simulink model "MATLAB_TEST"  (R2019b)
settings: Solver=FixedStepDiscrete  StartTime=0  StopTime=50  FixedStep=0.0025  RelTol=1e-3
undefined symbols (not defined in the file): BCM_COM_PROC_P20, BCM_COM_PROC_P20_SFW_R2018b, BCM_COM_PROC_P2_5, BCM_COM_PROC_P2_5_SFW_R2018b, BCM_COM_PROC_P5, BCM_COM_PROC_P5_SFW_R2018b, BCMA_ACCU_PT_Conf_Flt, BCMA_ACCU_PT_Unconf_Flt, BCMA_Antiskid_Off_Sanction, BCMA_Avionics_Conf_Flt, BCMA_BCM_CCDL_Conf_Flt, BCMA_BCM_CCDL_Unconf_Flt, BCMA_BCM_DBCU_INHIBITION_Conf_Flt, BCMA_BCM_DBCU_INHIBITION_Unconf_Flt, BCMA_BCP_ALT_Disp_Sw_Conf_Flt, BCMA_BCP_ALT_Disp_Sw_Unconf_Flt, BCMA_BCP_ALT_SW_ON_CMD_Conf_Flt, BCMA_BCP_ALT_SW_ON_CMD_Unconf_Flt, BCMA_BCP_PARK_OFF_SW_CMD_Conf_Flt, BCMA_BCP_PARK_OFF_SW_CMD_Unconf_Flt, BCMA_CF_BSELV_JCL, BCMA_CF_BSELV_JOP, BCMA_CF_BSELV_OC, BCMA_CF_BSELV_SC, BCMA_CF_LH_SV_JCL, BCMA_CF_LH_SV_JOP, BCMA_CF_LH_SV_OC, BCMA_CF_LH_SV_SC, BCMA_CF_PARK_BRK, BCMA_CF_RESIDUAL_PRESS, BCMA_CF_RH_SV_JCL, BCMA_CF_RH_SV_JOP, BCMA_CF_RH_SV_OC, BCMA_CF_RH_SV_SC, BCMA_CF_SELV_JCL, BCMA_CF_SELV_JOP, BCMA_CF_SELV_OC, BCMA_CF_SELV_SC, BCMA_CF_SV_DRIFT, BCMA_DBCU_ALT_MODE_Conf_Flt, BCMA_DBCU_ALT_MODE_Unconf_Flt, BCMA_DBCU_BRK_ORDER_FAIL_Conf_Flt, BCMA_DBCU_BRK_ORDER_FAIL_Unconf_Flt, BCMA_DBCU_Conf_Flt, BCMA_DBCU_DISPATCH_SW_ON_Conf_Flt, BCMA_DBCU_DISPATCH_SW_ON_Unconf_Flt, BCMA_DBCU_FAILED_Conf_Flt, BCMA_DBCU_FAILED_Unconf_Flt, BCMA_DFCS1_Capsule_Validity, BCMA_DFCS1_Label202_Corrupted, BCMA_DFCS1_Label202_Not_Refreshed, BCMA_DFCS1_Label204_Corrupted, BCMA_DFCS1_Label204_Not_Refreshed, BCMA_DFCS1_Label205_Corrupted, BCMA_DFCS1_Label205_Not_Refreshed, BCMA_DFCS1_Label206_Corrupted, BCMA_DFCS1_Label206_Not_Refreshed, BCMA_DFCS1_Label207_Corrupted, BCMA_DFCS1_Label207_Not_Refreshed, BCMA_DFCS3_Capsule_Validity ... (+762)
libraries: simulink x73, lib_MBD_Control x5
(part 7 of 16)

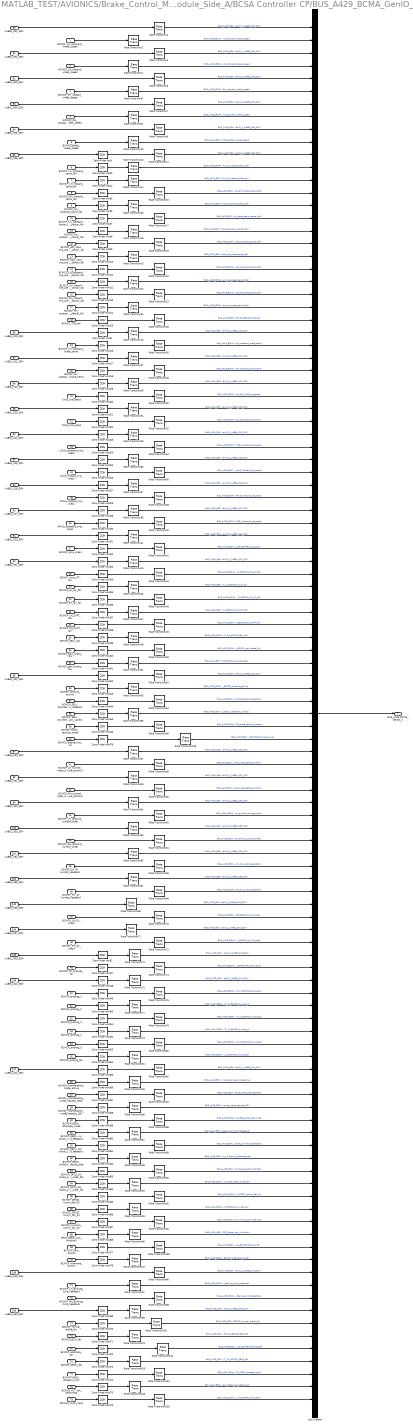
== system MATLAB_TEST/AVIONICS/Brake_Control_Module_Side_A/BCSA Controller CP/BUS_A429_BCMA_GenIO_2_TX ==
  BCMCP_LH_outboard_wheel_speed : Inport  OutDataTypeStr=single
  BCMCP_LH_inboard_wheel_speed : Inport  Port=2  OutDataTypeStr=single
  BCMCP_RH_inboard_wheel_speed : Inport  Port=3  OutDataTypeStr=single
  BCMCP_RH_outboard_wheel_speed : Inport  Port=4  OutDataTypeStr=single
  BCMCP_global_wheel_speed : Inport  Port=5  OutDataTypeStr=single
  BCMCP_LH_outboard_tacho_fail : Inport  Port=6  OutDataTypeStr=boolean
  BCMCP_LH_inboard_tacho_fail : Inport  Port=7  OutDataTypeStr=boolean
  BCMCP_RH_inboard_tacho_fail : Inport  Port=8  OutDataTypeStr=boolean
  BCMCP_RH_outboard_tacho_fail : Inport  Port=9  OutDataTypeStr=boolean
  BCMCP_LH_outboard_brake_temp_sensor_fail : Inport  Port=10  OutDataTypeStr=boolean
  BCMCP_RH_outboard_brake_temp_sensor_fail : Inport  Port=11  OutDataTypeStr=boolean
  BCMCP_left_nose_tire_press_sensor_fail : Inport  Port=12  OutDataTypeStr=boolean
  BCMCP_right_nose_tire_press_sensor_fail : Inport  Port=13  OutDataTypeStr=boolean
  BCMCP_LH_outboard_tire_press_sensor_fail : Inport  Port=14  OutDataTypeStr=boolean
  BCMCP_LH_inboard_tire_press_sensor_fail : Inport  Port=15  OutDataTypeStr=boolean
  BCMCP_RH_inboard_tire_press_sensor_fail : Inport  Port=16  OutDataTypeStr=boolean
  BCMCP_RH_outboard_tire_press_sensor_fail : Inport  Port=17  OutDataTypeStr=boolean
  BCMCP_TPIS_fail : Inport  Port=18  OutDataTypeStr=boolean
  BCMCP_LH_outboard_brake_temp : Inport  Port=19  OutDataTypeStr=single
  BCMCP_RH_outboard_brake_temp : Inport  Port=20  OutDataTypeStr=single
  LNLG_tire_press : Inport  Port=21  OutDataTypeStr=single
  RNLG_tire_press : Inport  Port=22  OutDataTypeStr=single
  LMLG_outboard_tire_press : Inport  Port=23  OutDataTypeStr=single
  LMLG_inboard_tire_press : Inport  Port=24  OutDataTypeStr=single
  RMLG_inboard_tire_press : Inport  Port=25  OutDataTypeStr=single
  RMLG_outboard_tire_press : Inport  Port=26  OutDataTypeStr=single
  BCMCP_accu_press : Inport  Port=27  OutDataTypeStr=single
  BCMCP_Accu_PT_fail : Inport  Port=28  OutDataTypeStr=boolean
  BCMCP_LH_SV_fail : Inport  Port=29  OutDataTypeStr=boolean
  BCMCP_RH_SV_fail : Inport  Port=30  OutDataTypeStr=boolean
  BCMCP_LH_SVPT_fail : Inport  Port=31  OutDataTypeStr=boolean
  BCMCP_RH_SVPT_fail : Inport  Port=32  OutDataTypeStr=boolean
  BCMCP_SELV_fail : Inport  Port=33  OutDataTypeStr=boolean
  BCMCP_park_brake_ON : Inport  Port=34  OutDataTypeStr=boolean
  BCMCP_park_brake_fail : Inport  Port=35  OutDataTypeStr=boolean
  BCMCP_antiskid_activity : Inport  Port=36  OutDataTypeStr=boolean
  BCMCP_SELV_discrete_status_readback : Inport  Port=37  OutDataTypeStr=boolean
  BCMCP_SELV_discrete_status_readback_validity : Inport  Port=38  OutDataTypeStr=boolean
  BCMCP_brake_residual_press : Inport  Port=39  OutDataTypeStr=boolean
  BCMCP_Engine_Run_Up : Inport  Port=40  OutDataTypeStr=boolean
  BCMCP_LH_current_order_before_antiskid : Inport  Port=41  OutDataTypeStr=single
  BCMCP_RH_current_order_before_antiskid : Inport  Port=42  OutDataTypeStr=single
  BCMCP_LH_antiskid_current_order : Inport  Port=43  OutDataTypeStr=single
  BCMCP_RH_antiskid_current_order : Inport  Port=44  OutDataTypeStr=single
  BCMCP_LH_SV_current_readback : Inport  Port=45  OutDataTypeStr=single
  BCMCP_RH_SV_current_readback : Inport  Port=46  OutDataTypeStr=single
  BCMCP_LH_SV_press : Inport  Port=47  OutDataTypeStr=single
  BCMCP_RH_SV_press : Inport  Port=48  OutDataTypeStr=single
  BCMCP_PP_channel_ID : Inport  Port=49
  BCMCP_pinprog_1 : Inport  Port=50  OutDataTypeStr=boolean
  BCMCP_pinprog_2 : Inport  Port=51  OutDataTypeStr=boolean
  BCMCP_pinprog_3 : Inport  Port=52  OutDataTypeStr=boolean
  BCMCP_pinprog_4 : Inport  Port=53  OutDataTypeStr=boolean
  BCMCP_pinprog_5 : Inport  Port=54  OutDataTypeStr=boolean
  BCMCP_pinprog_fail : Inport  Port=55  OutDataTypeStr=boolean
  BCMCP_maintenance_mode_active : Inport  Port=56  OutDataTypeStr=boolean
  BCMCP_maintenance_mode_request_GND : Inport  Port=57  OutDataTypeStr=boolean
  BCMCP_maintenance_mode_request_28V : Inport  Port=58  OutDataTypeStr=boolean
  BCMCP_DBCU_alternate_mode : Inport  Port=59  OutDataTypeStr=boolean
  BCMCP_DBCU_LH_brake_command_feedback : Inport  Port=60  OutDataTypeStr=boolean
  BCMCP_DBCU_RH_brake_command_feedback : Inport  Port=61  OutDataTypeStr=boolean
  BCMCP_DBCU_inhibition_opposite_side : Inport  Port=62  OutDataTypeStr=boolean
  BCMCP_DFCS_LH_brake_pedal_order_fail : Inport  Port=63  OutDataTypeStr=boolean
  BCMCP_DFCS_RH_brake_pedal_order_fail : Inport  Port=64  OutDataTypeStr=boolean
  BCMCP_DFCS1_comm_fail_RX : Inport  Port=65  OutDataTypeStr=boolean
  BCMCP_DFCS2_comm_fail_RX : Inport  Port=66  OutDataTypeStr=boolean
  BCMCP_Avionics_comm_fail_RX : Inport  Port=67  OutDataTypeStr=boolean
  DFCS_Decel_Law_Inhibition : Inport  Port=68  OutDataTypeStr=boolean
  BCMCP_Park_Switch : Inport  Port=69  OutDataTypeStr=boolean
  BCMCP_Alternate_Switch : Inport  Port=70  OutDataTypeStr=boolean
  BCMCP_LH_Braking_Cmd_Feedback : Inport  Port=71  OutDataTypeStr=single
  BCMCP_RH_Braking_Cmd_Feedback : Inport  Port=72  OutDataTypeStr=single
  BCMCP_normal_brake_fail : Inport  Port=73  OutDataTypeStr=boolean
  BCMCP_BCM_fail : Inport  Port=74  OutDataTypeStr=boolean
  BCMCP_alternate_fail : Inport  Port=75  OutDataTypeStr=boolean
  BCMCP_DBCU_fail : Inport  Port=76  OutDataTypeStr=boolean
  BCMCP_DBCU_dispatch_conf : Inport  Port=77  OutDataTypeStr=boolean
  BCMCP_PLT_not_performed : Inport  Port=78  OutDataTypeStr=boolean
  BCMCP_Minor_Fault : Inport  Port=79  OutDataTypeStr=boolean
  LABEL_001_SSM : Inport  Port=80
  LABEL_002_SSM : Inport  Port=81
  LABEL_003_SSM : Inport  Port=82
  LABEL_004_SSM : Inport  Port=83
  LABEL_005_SSM : Inport  Port=84
  LABEL_006_SSM : Inport  Port=85
  LABEL_010_SSM : Inport  Port=86
  LABEL_011_SSM : Inport  Port=87
  LABEL_012_SSM : Inport  Port=88
  LABEL_013_SSM : Inport  Port=89
  LABEL_014_SSM : Inport  Port=90
  LABEL_015_SSM : Inport  Port=91
  LABEL_016_SSM : Inport  Port=92
  LABEL_017_SSM : Inport  Port=93
  LABEL_020_SSM : Inport  Port=94
  LABEL_021_SSM : Inport  Port=95
  LABEL_022_SSM : Inport  Port=96
  LABEL_030_SSM : Inport  Port=97
  LABEL_031_SSM : Inport  Port=98
  LABEL_032_SSM : Inport  Port=99
  LABEL_033_SSM : Inport  Port=100
  LABEL_034_SSM : Inport  Port=101
  LABEL_035_SSM : Inport  Port=102
  LABEL_036_SSM : Inport  Port=103
  LABEL_037_SSM : Inport  Port=104
  LABEL_040_SSM : Inport  Port=105
  LABEL_041_SSM : Inport  Port=106
  LABEL_042_SSM : Inport  Port=107
  LABEL_043_SSM : Inport  Port=108
  LABEL_050_SSM : Inport  Port=109
  Bus Creator : BusCreator  Inputs=109  OutDataTypeStr=Bus: SMLK_BUS_A429_BCMA_GenIO_2  NonVirtualBus=on
      settings: InheritFromInputs=off
  Rate Transition{1..109} (109 alike) : RateTransition  Deterministic=off  OutPortSampleTime=1/50
      settings: AttributesFormatString=OutPortSampleTime %<OutPortSampleTime>
  Zero-Order Hold{,3..15,31..46,55..79} (55 alike) : ZeroOrderHold  SampleTime=0.08
      settings: AttributesFormatString=SampleTime %<SampleTime>
  Zero-Order Hold{1,16..30} (16 alike) : ZeroOrderHold  SampleTime=0.32
      settings: AttributesFormatString=SampleTime %<SampleTime>
  Zero-Order Hold{2,47..54} (9 alike) : ZeroOrderHold  SampleTime=1.28
      settings: AttributesFormatString=SampleTime %<SampleTime>
  BUS_A429_BCMA_GenIO_2 : Outport  VectorParamsAs1DForOutWhenUnconnected=off
  wires:
  Rate Transition34/1 -> Bus Creator/34  "BUS_A429_BCMA_GenIO_2_LABEL_014_LMLG_outboard_tire_press"
  Rate Transition33/1 -> Bus Creator/33  "BUS_A429_BCMA_GenIO_2_LABEL_014_SSM"
  Rate Transition35/1 -> Bus Creator/35  "BUS_A429_BCMA_GenIO_2_LABEL_015_SSM"
  Rate Transition36/1 -> Bus Creator/36  "BUS_A429_BCMA_GenIO_2_LABEL_015_LMLG_inboard_tire_press"
  Rate Transition37/1 -> Bus Creator/37  "BUS_A429_BCMA_GenIO_2_LABEL_016_SSM"
  Rate Transition38/1 -> Bus Creator/38  "BUS_A429_BCMA_GenIO_2_LABEL_016_RMLG_inboard_tire_press"
  Rate Transition32/1 -> Bus Creator/32  "BUS_A429_BCMA_GenIO_2_LABEL_013_RNLG_tire_press"
  Rate Transition39/1 -> Bus Creator/39  "BUS_A429_BCMA_GenIO_2_LABEL_017_SSM"
  Rate Transition11/1 -> Bus Creator/11  "BUS_A429_BCMA_GenIO_2_LABEL_006_SSM"
  Rate Transition14/1 -> Bus Creator/13  "BUS_A429_BCMA_GenIO_2_LABEL_006_DATA_BIT_12_BCMCP_LH_inboard_tacho_fail"
  Rate Transition30/1 -> Bus Creator/30  "BUS_A429_BCMA_GenIO_2_LABEL_012_LNLG_tire_press"
  Rate Transition40/1 -> Bus Creator/40  "BUS_A429_BCMA_GenIO_2_LABEL_017_RMLG_outboard_tire_press"
  Rate Transition15/1 -> Bus Creator/14  "BUS_A429_BCMA_GenIO_2_LABEL_006_DATA_BIT_13_BCMCP_RH_inboard_tacho_fail"
  Rate Transition16/1 -> Bus Creator/15  "BUS_A429_BCMA_GenIO_2_LABEL_006_DATA_BIT_14_BCMCP_RH_outboard_tacho_fail"
  Rate Transition17/1 -> Bus Creator/16  "BUS_A429_BCMA_GenIO_2_LABEL_006_DATA_BIT_15_BCMCP_LH_outboard_brake_temp_sensor_fail"
  Rate Transition29/1 -> Bus Creator/29  "BUS_A429_BCMA_GenIO_2_LABEL_012_SSM"
  Rate Transition28/1 -> Bus Creator/28  "BUS_A429_BCMA_GenIO_2_LABEL_011_BCMCP_RH_outboard_brake_temp"
  Rate Transition19/1 -> Bus Creator/18  "BUS_A429_BCMA_GenIO_2_LABEL_006_DATA_BIT_17_BCMCP_left_nose_tire_press_sensor_fail"
  Rate Transition20/1 -> Bus Creator/19  "BUS_A429_BCMA_GenIO_2_LABEL_006_DATA_BIT_18_BCMCP_right_nose_tire_press_sensor_fail"
  Rate Transition55/1 -> Bus Creator/55  "BUS_A429_BCMA_GenIO_2_LABEL_022_DATA_BIT_13_BCMCP_SELV_discrete_status_readback_validity"
  Rate Transition56/1 -> Bus Creator/56  "BUS_A429_BCMA_GenIO_2_LABEL_022_DATA_BIT_14_BCMCP_brake_residual_press"
  Rate Transition10/1 -> Bus Creator/10  "BUS_A429_BCMA_GenIO_2_LABEL_005_BCMCP_global_wheel_speed"
  Rate Transition21/1 -> Bus Creator/20  "BUS_A429_BCMA_GenIO_2_LABEL_006_DATA_BIT_19_BCMCP_LH_outboard_tire_press_sensor_fail"
  Rate Transition27/1 -> Bus Creator/27  "BUS_A429_BCMA_GenIO_2_LABEL_011_SSM"
  Rate Transition41/1 -> Bus Creator/41  "BUS_A429_BCMA_GenIO_2_LABEL_020_SSM"
  Rate Transition50/1 -> Bus Creator/50  "BUS_A429_BCMA_GenIO_2_LABEL_021_DATA_BIT_17_BCMCP_park_brake_ON"
  Rate Transition51/1 -> Bus Creator/51  "BUS_A429_BCMA_GenIO_2_LABEL_021_DATA_BIT_18_BCMCP_park_brake_fail"
  Rate Transition54/1 -> Bus Creator/54  "BUS_A429_BCMA_GenIO_2_LABEL_022_DATA_BIT_12_BCMCP_SELV_discrete_status_readback"
  Rate Transition9/1 -> Bus Creator/9  "BUS_A429_BCMA_GenIO_2_LABEL_005_SSM"
  Rate Transition42/1 -> Bus Creator/42  "BUS_A429_BCMA_GenIO_2_LABEL_020_BCMCP_accu_press"
  Rate Transition43/1 -> Bus Creator/43  "BUS_A429_BCMA_GenIO_2_LABEL_021_SSM"
  Rate Transition45/1 -> Bus Creator/45  "BUS_A429_BCMA_GenIO_2_LABEL_021_DATA_BIT_12_BCMCP_LH_SV_fail"
  Rate Transition46/1 -> Bus Creator/46  "BUS_A429_BCMA_GenIO_2_LABEL_021_DATA_BIT_13_BCMCP_RH_SV_fail"
  Rate Transition47/1 -> Bus Creator/47  "BUS_A429_BCMA_GenIO_2_LABEL_021_DATA_BIT_14_BCMCP_LH_SVPT_fail"
  Rate Transition48/1 -> Bus Creator/48  "BUS_A429_BCMA_GenIO_2_LABEL_021_DATA_BIT_15_BCMCP_RH_SVPT_fail"
  Rate Transition49/1 -> Bus Creator/49  "BUS_A429_BCMA_GenIO_2_LABEL_021_DATA_BIT_16_BCMCP_SELV_fail"
  Rate Transition26/1 -> Bus Creator/26  "BUS_A429_BCMA_GenIO_2_LABEL_010_BCMCP_LH_outboard_brake_temp"
  Rate Transition44/1 -> Bus Creator/44  "BUS_A429_BCMA_GenIO_2_LABEL_021_DATA_BIT_11_BCMCP_Accu_PT_fail"
  Rate Transition52/1 -> Bus Creator/52  "BUS_A429_BCMA_GenIO_2_LABEL_022_SSM"
  Rate Transition8/1 -> Bus Creator/8  "BUS_A429_BCMA_GenIO_2_LABEL_004_BCMCP_RH_outboard_wheel_speed"
  Rate Transition23/1 -> Bus Creator/22  "BUS_A429_BCMA_GenIO_2_LABEL_006_DATA_BIT_21_BCMCP_RH_inboard_tire_press_sensor_fail"
  Rate Transition13/1 -> Bus Creator/25  "BUS_A429_BCMA_GenIO_2_LABEL_010_SSM"
  Rate Transition53/1 -> Bus Creator/53  "BUS_A429_BCMA_GenIO_2_LABEL_022_DATA_BIT_11_BCMCP_antiskid_activity"
  Rate Transition24/1 -> Bus Creator/23  "BUS_A429_BCMA_GenIO_2_LABEL_006_DATA_BIT_22_BCMCP_RH_outboard_tire_press_sensor_fail"
  Rate Transition25/1 -> Bus Creator/24  "BUS_A429_BCMA_GenIO_2_LABEL_006_DATA_BIT_23_BCMCP_TPIS_fail"
  Rate Transition7/1 -> Bus Creator/7  "BUS_A429_BCMA_GenIO_2_LABEL_004_SSM"
  Rate Transition95/1 -> Bus Creator/96  "BUS_A429_BCMA_GenIO_2_LABEL_042_DATA_BIT_23_DFCS_Decel_Law_Inhibition"
  Rate Transition93/1 -> Bus Creator/94  "BUS_A429_BCMA_GenIO_2_LABEL_042_DATA_BIT_21_BCMCP_DFCS2_comm_fail_RX"
  Rate Transition94/1 -> Bus Creator/95  "BUS_A429_BCMA_GenIO_2_LABEL_042_DATA_BIT_22_BCMCP_Avionics_comm_fail_RX"
  Rate Transition6/1 -> Bus Creator/6  "BUS_A429_BCMA_GenIO_2_LABEL_003_BCMCP_RH_inboard_wheel_speed"
  Rate Transition92/1 -> Bus Creator/93  "BUS_A429_BCMA_GenIO_2_LABEL_042_DATA_BIT_20_BCMCP_DFCS1_comm_fail_RX"
  Rate Transition96/1 -> Bus Creator/99  "BUS_A429_BCMA_GenIO_2_LABEL_043_SSM"
  Rate Transition91/1 -> Bus Creator/92  "BUS_A429_BCMA_GenIO_2_LABEL_042_DATA_BIT_19_BCMCP_DFCS_RH_brake_pedal_order_fail"
  Rate Transition98/1 -> Bus Creator/101  "BUS_A429_BCMA_GenIO_2_LABEL_043_BCMCP_RH_Braking_Cmd_Feedback"
  Rate Transition5/1 -> Bus Creator/5  "BUS_A429_BCMA_GenIO_2_LABEL_003_SSM"
  Rate Transition90/1 -> Bus Creator/91  "BUS_A429_BCMA_GenIO_2_LABEL_042_DATA_BIT_18_BCMCP_DFCS_LH_brake_pedal_order_fail"
  Rate Transition97/1 -> Bus Creator/100  "BUS_A429_BCMA_GenIO_2_LABEL_043_BCMCP_LH_Braking_Cmd_Feedback"
  Rate Transition89/1 -> Bus Creator/90  "BUS_A429_BCMA_GenIO_2_LABEL_042_DATA_BIT_17_BCMCP_DBCU_inhibition_opposite_side"
  Rate Transition87/1 -> Bus Creator/88  "BUS_A429_BCMA_GenIO_2_LABEL_042_DATA_BIT_15_BCMCP_DBCU_LH_brake_command_feedback"
  Rate Transition105/1 -> Bus Creator/108  "BUS_A429_BCMA_GenIO_2_LABEL_050_DATA_BIT_16_BCMCP_Brake_Tests_not_performed"
  Rate Transition88/1 -> Bus Creator/89  "BUS_A429_BCMA_GenIO_2_LABEL_042_DATA_BIT_16_BCMCP_DBCU_RH_brake_command_feedback"
  Rate Transition99/1 -> Bus Creator/102  "BUS_A429_BCMA_GenIO_2_LABEL_050_SSM"
  Rate Transition104/1 -> Bus Creator/107  "BUS_A429_BCMA_GenIO_2_LABEL_050_DATA_BIT_15_BCMCP_DBCU_dispatch_conf"
  Rate Transition86/1 -> Bus Creator/87  "BUS_A429_BCMA_GenIO_2_LABEL_042_DATA_BIT_14_BCMCP_DBCU_alternate_mode"
  Rate Transition103/1 -> Bus Creator/106  "BUS_A429_BCMA_GenIO_2_LABEL_050_DATA_BIT_14_BCMCP_DBCU_fail"
  Rate Transition85/1 -> Bus Creator/86  "BUS_A429_BCMA_GenIO_2_LABEL_042_DATA_BIT_13_BCMCP_maintenance_mode_request_28V"
  Rate Transition4/1 -> Bus Creator/4  "BUS_A429_BCMA_GenIO_2_LABEL_002_BCMCP_LH_inboard_wheel_speed"
  Rate Transition80/1 -> Bus Creator/81  "BUS_A429_BCMA_GenIO_2_LABEL_041_DATA_BIT_15_BCMCP_pinprog_5"
  Rate Transition81/1 -> Bus Creator/82  "BUS_A429_BCMA_GenIO_2_LABEL_041_DATA_BIT_16_BCMCP_pinprog_fail"
  Rate Transition82/1 -> Bus Creator/83  "BUS_A429_BCMA_GenIO_2_LABEL_042_SSM"
  Rate Transition84/1 -> Bus Creator/85  "BUS_A429_BCMA_GenIO_2_LABEL_042_DATA_BIT_12_BCMCP_maintenance_mode_request_GND"
  Rate Transition100/1 -> Bus Creator/103  "BUS_A429_BCMA_GenIO_2_LABEL_050_DATA_BIT_11_BCMCP_normal_brake_fail"
  Rate Transition102/1 -> Bus Creator/105  "BUS_A429_BCMA_GenIO_2_LABEL_050_DATA_BIT_13_BCMCP_alternate_fail"
  Rate Transition83/1 -> Bus Creator/84  "BUS_A429_BCMA_GenIO_2_LABEL_042_DATA_BIT_11_BCMCP_maintenance_mode_active"
  Rate Transition101/1 -> Bus Creator/104  "BUS_A429_BCMA_GenIO_2_LABEL_050_DATA_BIT_12_BCMCP_BCM_fail"
  Rate Transition3/1 -> Bus Creator/3  "BUS_A429_BCMA_GenIO_2_LABEL_002_SSM"
  Rate Transition2/1 -> Bus Creator/2  "BUS_A429_BCMA_GenIO_2_LABEL_001_BCMCP_LH_outboard_wheel_speed"
  Rate Transition1/1 -> Bus Creator/1  "BUS_A429_BCMA_GenIO_2_LABEL_001_SSM"
  Rate Transition22/1 -> Bus Creator/21  "BUS_A429_BCMA_GenIO_2_LABEL_006_DATA_BIT_20_BCMCP_LH_inboard_tire_press_sensor_fail"
  Rate Transition31/1 -> Bus Creator/31  "BUS_A429_BCMA_GenIO_2_LABEL_013_SSM"
  Bus Creator/1 -> BUS_A429_BCMA_GenIO_2/1
  Rate Transition12/1 -> Bus Creator/12  "BUS_A429_BCMA_GenIO_2_LABEL_006_DATA_BIT_11_BCMCP_LH_outboard_tacho_fail"
  LABEL_001_SSM/1 -> Rate Transition1/1
  BCMCP_LH_outboard_wheel_speed/1 -> Rate Transition2/1
  LABEL_002_SSM/1 -> Rate Transition3/1
  BCMCP_LH_inboard_wheel_speed/1 -> Rate Transition4/1
  LABEL_003_SSM/1 -> Rate Transition5/1
  BCMCP_RH_inboard_wheel_speed/1 -> Rate Transition6/1
  LABEL_004_SSM/1 -> Rate Transition7/1
  BCMCP_RH_outboard_wheel_speed/1 -> Rate Transition8/1
  LABEL_005_SSM/1 -> Rate Transition9/1
  BCMCP_global_wheel_speed/1 -> Rate Transition10/1
  LABEL_006_SSM/1 -> Zero-Order Hold/1
  BCMCP_LH_outboard_tacho_fail/1 -> Zero-Order Hold3/1
  BCMCP_LH_inboard_tacho_fail/1 -> Zero-Order Hold4/1
  BCMCP_RH_inboard_tacho_fail/1 -> Zero-Order Hold5/1
  BCMCP_RH_outboard_tacho_fail/1 -> Zero-Order Hold6/1
  BCMCP_LH_outboard_brake_temp_sensor_fail/1 -> Zero-Order Hold7/1
  BCMCP_RH_outboard_brake_temp_sensor_fail/1 -> Zero-Order Hold8/1
  BCMCP_left_nose_tire_press_sensor_fail/1 -> Zero-Order Hold9/1
  BCMCP_right_nose_tire_press_sensor_fail/1 -> Zero-Order Hold10/1
  BCMCP_LH_outboard_tire_press_sensor_fail/1 -> Zero-Order Hold11/1
  BCMCP_LH_inboard_tire_press_sensor_fail/1 -> Zero-Order Hold12/1
  BCMCP_RH_inboard_tire_press_sensor_fail/1 -> Zero-Order Hold13/1
  BCMCP_RH_outboard_tire_press_sensor_fail/1 -> Zero-Order Hold14/1
  BCMCP_TPIS_fail/1 -> Zero-Order Hold15/1
  LABEL_010_SSM/1 -> Zero-Order Hold1/1
  BCMCP_LH_outboard_brake_temp/1 -> Zero-Order Hold16/1
  LABEL_011_SSM/1 -> Zero-Order Hold17/1
  BCMCP_RH_outboard_brake_temp/1 -> Zero-Order Hold18/1
  LABEL_012_SSM/1 -> Zero-Order Hold19/1
  LNLG_tire_press/1 -> Zero-Order Hold20/1
  LABEL_013_SSM/1 -> Zero-Order Hold21/1
  RNLG_tire_press/1 -> Zero-Order Hold22/1
  LABEL_014_SSM/1 -> Zero-Order Hold23/1
  LMLG_outboard_tire_press/1 -> Zero-Order Hold24/1
  LABEL_015_SSM/1 -> Zero-Order Hold25/1
  LMLG_inboard_tire_press/1 -> Zero-Order Hold26/1
  LABEL_016_SSM/1 -> Zero-Order Hold27/1
  RMLG_inboard_tire_press/1 -> Zero-Order Hold28/1
  LABEL_017_SSM/1 -> Zero-Order Hold29/1
  RMLG_outboard_tire_press/1 -> Zero-Order Hold30/1
  LABEL_020_SSM/1 -> Zero-Order Hold31/1
  BCMCP_accu_press/1 -> Zero-Order Hold32/1
  LABEL_021_SSM/1 -> Zero-Order Hold33/1
  BCMCP_Accu_PT_fail/1 -> Zero-Order Hold34/1
  BCMCP_LH_SV_fail/1 -> Zero-Order Hold35/1
  BCMCP_RH_SV_fail/1 -> Zero-Order Hold36/1
  BCMCP_LH_SVPT_fail/1 -> Zero-Order Hold37/1
  BCMCP_RH_SVPT_fail/1 -> Zero-Order Hold38/1
  BCMCP_SELV_fail/1 -> Zero-Order Hold39/1
  BCMCP_park_brake_ON/1 -> Zero-Order Hold40/1
  BCMCP_park_brake_fail/1 -> Zero-Order Hold41/1
  LABEL_022_SSM/1 -> Zero-Order Hold42/1
  BCMCP_antiskid_activity/1 -> Zero-Order Hold43/1
  BCMCP_SELV_discrete_status_readback/1 -> Zero-Order Hold44/1
  BCMCP_SELV_discrete_status_readback_validity/1 -> Zero-Order Hold45/1
  BCMCP_brake_residual_press/1 -> Zero-Order Hold46/1
  LABEL_030_SSM/1 -> Rate Transition57/1
  BCMCP_LH_current_order_before_antiskid/1 -> Rate Transition58/1
  LABEL_031_SSM/1 -> Rate Transition59/1
  BCMCP_RH_current_order_before_antiskid/1 -> Rate Transition60/1
  LABEL_032_SSM/1 -> Rate Transition61/1
  BCMCP_LH_antiskid_current_order/1 -> Rate Transition62/1
  LABEL_033_SSM/1 -> Rate Transition63/1
  BCMCP_RH_antiskid_current_order/1 -> Rate Transition64/1
  LABEL_034_SSM/1 -> Rate Transition65/1
  BCMCP_LH_SV_current_readback/1 -> Rate Transition66/1
  LABEL_035_SSM/1 -> Rate Transition67/1
  BCMCP_RH_SV_current_readback/1 -> Rate Transition68/1
  LABEL_036_SSM/1 -> Rate Transition69/1
  BCMCP_LH_SV_press/1 -> Rate Transition70/1
  LABEL_037_SSM/1 -> Rate Transition71/1
  BCMCP_RH_SV_press/1 -> Rate Transition72/1
  LABEL_040_SSM/1 -> Zero-Order Hold2/1
  BCMCP_PP_channel_ID/1 -> Zero-Order Hold47/1
  LABEL_041_SSM/1 -> Zero-Order Hold48/1
  BCMCP_pinprog_1/1 -> Zero-Order Hold49/1
  BCMCP_pinprog_2/1 -> Zero-Order Hold50/1
  BCMCP_pinprog_3/1 -> Zero-Order Hold51/1
  BCMCP_pinprog_4/1 -> Zero-Order Hold52/1
  BCMCP_pinprog_5/1 -> Zero-Order Hold53/1
  BCMCP_pinprog_fail/1 -> Zero-Order Hold54/1
  LABEL_042_SSM/1 -> Zero-Order Hold55/1
  BCMCP_maintenance_mode_active/1 -> Zero-Order Hold56/1
  BCMCP_maintenance_mode_request_GND/1 -> Zero-Order Hold57/1
  BCMCP_maintenance_mode_request_28V/1 -> Zero-Order Hold58/1
  BCMCP_DBCU_alternate_mode/1 -> Zero-Order Hold59/1
  BCMCP_DBCU_LH_brake_command_feedback/1 -> Zero-Order Hold60/1
  BCMCP_DBCU_RH_brake_command_feedback/1 -> Zero-Order Hold61/1
  BCMCP_DBCU_inhibition_opposite_side/1 -> Zero-Order Hold62/1
  BCMCP_DFCS_LH_brake_pedal_order_fail/1 -> Zero-Order Hold63/1
  BCMCP_DFCS_RH_brake_pedal_order_fail/1 -> Zero-Order Hold64/1
  BCMCP_DFCS1_comm_fail_RX/1 -> Zero-Order Hold65/1
  BCMCP_DFCS2_comm_fail_RX/1 -> Zero-Order Hold66/1
  BCMCP_Avionics_comm_fail_RX/1 -> Zero-Order Hold67/1
  DFCS_Decel_Law_Inhibition/1 -> Zero-Order Hold68/1
  LABEL_043_SSM/1 -> Rate Transition96/1
  BCMCP_LH_Braking_Cmd_Feedback/1 -> Rate Transition97/1
  BCMCP_RH_Braking_Cmd_Feedback/1 -> Rate Transition98/1
  LABEL_050_SSM/1 -> Zero-Order Hold69/1
  BCMCP_normal_brake_fail/1 -> Zero-Order Hold70/1
  BCMCP_BCM_fail/1 -> Zero-Order Hold71/1
  BCMCP_alternate_fail/1 -> Zero-Order Hold72/1
  BCMCP_DBCU_fail/1 -> Zero-Order Hold73/1
  BCMCP_DBCU_dispatch_conf/1 -> Zero-Order Hold74/1
  BCMCP_PLT_not_performed/1 -> Zero-Order Hold75/1
  Rate Transition18/1 -> Bus Creator/17  "BUS_A429_BCMA_GenIO_2_LABEL_006_DATA_BIT_16_BCMCP_RH_outboard_brake_temp_sensor_fail"
  Zero-Order Hold/1 -> Rate Transition11/1
  Zero-Order Hold1/1 -> Rate Transition13/1
  Zero-Order Hold2/1 -> Rate Transition73/1
  Zero-Order Hold3/1 -> Rate Transition12/1
  Zero-Order Hold4/1 -> Rate Transition14/1
  Zero-Order Hold5/1 -> Rate Transition15/1
  Zero-Order Hold6/1 -> Rate Transition16/1
  Zero-Order Hold7/1 -> Rate Transition17/1
  Zero-Order Hold8/1 -> Rate Transition18/1
  Zero-Order Hold9/1 -> Rate Transition19/1
  Zero-Order Hold10/1 -> Rate Transition20/1
  Zero-Order Hold11/1 -> Rate Transition21/1
  Zero-Order Hold12/1 -> Rate Transition22/1
  Zero-Order Hold13/1 -> Rate Transition23/1
  Zero-Order Hold14/1 -> Rate Transition24/1
  Zero-Order Hold15/1 -> Rate Transition25/1
  Zero-Order Hold16/1 -> Rate Transition26/1
  Zero-Order Hold17/1 -> Rate Transition27/1
  Zero-Order Hold18/1 -> Rate Transition28/1
  Zero-Order Hold19/1 -> Rate Transition29/1
  Zero-Order Hold20/1 -> Rate Transition30/1
  Zero-Order Hold21/1 -> Rate Transition31/1
  Zero-Order Hold22/1 -> Rate Transition32/1
  Zero-Order Hold23/1 -> Rate Transition33/1
  Zero-Order Hold24/1 -> Rate Transition34/1
  Zero-Order Hold25/1 -> Rate Transition35/1
  Zero-Order Hold26/1 -> Rate Transition36/1
  Zero-Order Hold27/1 -> Rate Transition37/1
  Zero-Order Hold28/1 -> Rate Transition38/1
  Zero-Order Hold29/1 -> Rate Transition39/1
  Zero-Order Hold30/1 -> Rate Transition40/1
  Zero-Order Hold31/1 -> Rate Transition41/1
  Zero-Order Hold32/1 -> Rate Transition42/1
  Zero-Order Hold33/1 -> Rate Transition43/1
  Zero-Order Hold34/1 -> Rate Transition44/1
  Zero-Order Hold35/1 -> Rate Transition45/1
  Zero-Order Hold36/1 -> Rate Transition46/1
  Zero-Order Hold37/1 -> Rate Transition47/1
  Zero-Order Hold38/1 -> Rate Transition48/1
  Zero-Order Hold39/1 -> Rate Transition49/1
  Zero-Order Hold40/1 -> Rate Transition50/1
  Zero-Order Hold41/1 -> Rate Transition51/1
  Zero-Order Hold42/1 -> Rate Transition52/1
  Zero-Order Hold43/1 -> Rate Transition53/1
  Zero-Order Hold44/1 -> Rate Transition54/1
  Zero-Order Hold45/1 -> Rate Transition55/1
  Zero-Order Hold46/1 -> Rate Transition56/1
  Zero-Order Hold47/1 -> Rate Transition74/1
  Zero-Order Hold48/1 -> Rate Transition75/1
  Zero-Order Hold49/1 -> Rate Transition76/1
  Zero-Order Hold50/1 -> Rate Transition77/1
  Zero-Order Hold51/1 -> Rate Transition78/1
  Zero-Order Hold52/1 -> Rate Transition79/1
  Zero-Order Hold53/1 -> Rate Transition80/1
  Zero-Order Hold54/1 -> Rate Transition81/1
  Zero-Order Hold55/1 -> Rate Transition82/1
  Zero-Order Hold56/1 -> Rate Transition83/1
  Zero-Order Hold57/1 -> Rate Transition84/1
  Zero-Order Hold58/1 -> Rate Transition85/1
  Zero-Order Hold59/1 -> Rate Transition86/1
  Zero-Order Hold60/1 -> Rate Transition87/1
  Zero-Order Hold61/1 -> Rate Transition88/1
  Zero-Order Hold62/1 -> Rate Transition89/1
  Zero-Order Hold63/1 -> Rate Transition90/1
  Zero-Order Hold64/1 -> Rate Transition91/1
  Zero-Order Hold65/1 -> Rate Transition92/1
  Zero-Order Hold66/1 -> Rate Transition93/1
  Zero-Order Hold67/1 -> Rate Transition94/1
  Zero-Order Hold68/1 -> Rate Transition95/1
  Zero-Order Hold69/1 -> Rate Transition99/1
  Zero-Order Hold70/1 -> Rate Transition100/1
  Zero-Order Hold71/1 -> Rate Transition101/1
  Zero-Order Hold72/1 -> Rate Transition102/1
  Zero-Order Hold73/1 -> Rate Transition103/1
  Zero-Order Hold74/1 -> Rate Transition104/1
  Zero-Order Hold75/1 -> Rate Transition105/1
  Zero-Order Hold76/1 -> Rate Transition106/1
  Rate Transition106/1 -> Bus Creator/109  "BUS_A429_BCMA_GenIO_2_LABEL_050_DATA_BIT_17_BCMCP_Minor_Fault"
  BCMCP_Minor_Fault/1 -> Zero-Order Hold76/1
  Rate Transition107/1 -> Bus Creator/98  "BUS_A429_BCMA_GenIO_2_LABEL_042_DATA_BIT_25_BCMCP_Alternate_Switch"
  Rate Transition108/1 -> Bus Creator/97  "BUS_A429_BCMA_GenIO_2_LABEL_042_DATA_BIT_24_BCMCP_Park_Switch"
  BCMCP_Alternate_Switch/1 -> Zero-Order Hold78/1
  BCMCP_Park_Switch/1 -> Zero-Order Hold77/1
  Zero-Order Hold77/1 -> Rate Transition108/1
  Zero-Order Hold78/1 -> Rate Transition107/1
  Rate Transition79/1 -> Bus Creator/80  "BUS_A429_BCMA_GenIO_2_LABEL_041_DATA_BIT_14_BCMCP_pinprog_4"
  Rate Transition78/1 -> Bus Creator/79  "BUS_A429_BCMA_GenIO_2_LABEL_041_DATA_BIT_13_BCMCP_pinprog_3"
  Rate Transition109/1 -> Bus Creator/57  "BUS_A429_BCMA_GenIO_2_LABEL_022_DATA_BIT_15_BCMCP_Engine_Run_Up"
  Rate Transition58/1 -> Bus Creator/59  "BUS_A429_BCMA_GenIO_2_LABEL_030_BCMCP_LH_current_order_before_antiskid"
  Rate Transition60/1 -> Bus Creator/61  "BUS_A429_BCMA_GenIO_2_LABEL_031_BCMCP_RH_current_order_before_antiskid"
  Rate Transition62/1 -> Bus Creator/63  "BUS_A429_BCMA_GenIO_2_LABEL_032_BCMCP_LH_antiskid_current_order"
  Rate Transition64/1 -> Bus Creator/65  "BUS_A429_BCMA_GenIO_2_LABEL_033_BCMCP_RH_antiskid_current_order"
  Rate Transition66/1 -> Bus Creator/67  "BUS_A429_BCMA_GenIO_2_LABEL_034_BCMCP_LH_SV_current_readback"
  Rate Transition68/1 -> Bus Creator/69  "BUS_A429_BCMA_GenIO_2_LABEL_035_BCMCP_RH_SV_current_readback"
  Rate Transition70/1 -> Bus Creator/71  "BUS_A429_BCMA_GenIO_2_LABEL_036_BCMCP_LH_SV_press"
  Rate Transition72/1 -> Bus Creator/73  "BUS_A429_BCMA_GenIO_2_LABEL_037_BCMCP_RH_SV_press"
  Rate Transition74/1 -> Bus Creator/75  "BUS_A429_BCMA_GenIO_2_LABEL_040_BCMCP_PP_channel_ID"
  Rate Transition76/1 -> Bus Creator/77  "BUS_A429_BCMA_GenIO_2_LABEL_041_DATA_BIT_11_BCMCP_pinprog_1"
  Rate Transition73/1 -> Bus Creator/74  "BUS_A429_BCMA_GenIO_2_LABEL_040_SSM"
  Rate Transition75/1 -> Bus Creator/76  "BUS_A429_BCMA_GenIO_2_LABEL_041_SSM"
  Rate Transition77/1 -> Bus Creator/78  "BUS_A429_BCMA_GenIO_2_LABEL_041_DATA_BIT_12_BCMCP_pinprog_2"
  Rate Transition57/1 -> Bus Creator/58  "BUS_A429_BCMA_GenIO_2_LABEL_030_SSM"
  Rate Transition59/1 -> Bus Creator/60  "BUS_A429_BCMA_GenIO_2_LABEL_031_SSM"
  Rate Transition61/1 -> Bus Creator/62  "BUS_A429_BCMA_GenIO_2_LABEL_032_SSM"
  Rate Transition63/1 -> Bus Creator/64  "BUS_A429_BCMA_GenIO_2_LABEL_033_SSM"
  Rate Transition65/1 -> Bus Creator/66  "BUS_A429_BCMA_GenIO_2_LABEL_034_SSM"
  Rate Transition67/1 -> Bus Creator/68  "BUS_A429_BCMA_GenIO_2_LABEL_035_SSM"
  Rate Transition69/1 -> Bus Creator/70  "BUS_A429_BCMA_GenIO_2_LABEL_036_SSM"
  Rate Transition71/1 -> Bus Creator/72  "BUS_A429_BCMA_GenIO_2_LABEL_037_SSM"
  Zero-Order Hold79/1 -> Rate Transition109/1
  BCMCP_Engine_Run_Up/1 -> Zero-Order Hold79/1

== system MATLAB_TEST/AVIONICS/Brake_Control_Module_Side_A/BCSA Controller CP/BUS_CAN_BCM_CCDL_RX_ ==
  BUS_CAN_BCM_CCDL_RX : Inport
  Bus Selector : BusSelector  OutputSignals=BUS_CAN_BCM_CCDL_TX_V_BCM_COM_Big_Gamma_Trig_Out_W1,BUS_CAN_BCM_CCDL_TX_V_BCM_COM_Big_Gamma_Trig_Out_W2,BUS_CAN_BCM_CCDL_TX_V_BCM_COM_Big_Gamma_Trig_Out_W3,BUS_CAN_BCM_CCDL_TX_V_BCM_COM_Big_Gamma_Trig_Out_W4,BUS_CAN_BCM_CCDL_TX_V_BCM_COM_Big_Slip_Trig_Out_W1,BUS_CAN_BCM_CCDL_TX_V_BCM_COM_Big_Slip_Trig_Out_W2,BUS_CAN_BCM_CCDL_TX_V_BCM_COM_Big_Slip_Trig_Out_W3,BUS_CAN_BCM_CCDL_TX_V_BCM_COM_Big_Slip_Trig_Out_W4,BUS_CAN_BCM_CCDL_TX_V_BCM_COM_Big_Slip_WD_Trig_Out_W1,BUS_CAN_BCM_CCDL_TX_V_BCM_COM_Big_Slip_WD_Trig_Out_W2,BUS_CAN_BCM_CCDL_TX_V_BCM_COM_Big_Slip_WD_Trig_Out_W3,BUS_CAN_BCM_CCDL_TX_V_BCM_COM_Big_Slip_WD_Trig_Out_W4,BUS_CAN_BCM_CCDL_TX_V_BCM_COM_Small_Slip_Trig_Out_W1,BUS_CAN_BCM_CCDL_TX_V_BCM_COM_Small_Slip_Trig_Out_W2,BUS_CAN_BCM_CCDL_TX_V_BCM_COM_Small_Slip_Trig_Out_W3,BUS_CAN_BCM_CCDL_TX_V_BCM_COM_Small_Slip_Trig_Out_W4,BUS_CAN_BCM_CCDL_TX_V_BCM_COM_Target_Speed_Out_W1,BUS_CAN_BCM_CCDL_TX_V_BCM_COM_Target_Speed_Out_W2,BUS_CAN_BCM_CCDL_TX_V_BCM_COM_Target_Speed_Out_W3,BUS_CAN_BCM_CCDL_TX_V_BCM_COM_Target_Speed_Out_W4,BUS_CAN_BCM_CCDL_TX_V_BCM_COM_Adhesion_Out_W1,BUS_CAN_BCM_CCDL_TX_V_BCM_COM_Adhesion_Out_W2,BUS_CAN_BCM_CCDL_TX_V_BCM_COM_Adhesion_Out_W3,BUS_CAN_BCM_CCDL_TX_V_BCM_COM_Adhesion_Out_W4,BUS_CAN_BCM_CCDL_TX_V_BCM_COM_Opt_Adhesion_Out_W1,BUS_CAN_BCM_CCDL_TX_V_BCM_COM_Opt_Adhesion_Out_W2,BUS_CAN_BCM_CCDL_TX_V_BCM_COM_Opt_Adhesion_Out_W3,BUS_CAN_BCM_CCDL_TX_V_BCM_COM_Opt_Adhesion_Out_W4
  Mux{,1..13} (14 alike) : Mux  Inputs=2
  V_BCM_COM_Big_Gamma_Trig_Out_W12 : Outport  VectorParamsAs1DForOutWhenUnconnected=off
  V_BCM_COM_Big_Gamma_Trig_Out_W34 : Outport  Port=2  VectorParamsAs1DForOutWhenUnconnected=off
  V_BCM_COM_Big_Slip_Trig_Out_W12 : Outport  Port=3  VectorParamsAs1DForOutWhenUnconnected=off
  V_BCM_COM_Big_Slip_Trig_Out_W34 : Outport  Port=4  VectorParamsAs1DForOutWhenUnconnected=off
  V_BCM_COM_Big_Slip_WD_In_Mon_W12 : Outport  Port=5  VectorParamsAs1DForOutWhenUnconnected=off
  V_BCM_COM_Big_Slip_WD_In_Mon_W34 : Outport  Port=6  VectorParamsAs1DForOutWhenUnconnected=off
  V_BCM_COM_Small_Slip_Trig_Out_W12 : Outport  Port=7  VectorParamsAs1DForOutWhenUnconnected=off
  V_BCM_COM_Small_Slip_Trig_Out_W34 : Outport  Port=8  VectorParamsAs1DForOutWhenUnconnected=off
  V_BCM_COM_Target_Speed_Out_W12 : Outport  Port=9  VectorParamsAs1DForOutWhenUnconnected=off
  V_BCM_COM_Target_Speed_Out_W34 : Outport  Port=10  VectorParamsAs1DForOutWhenUnconnected=off
  V_BCM_COM_Adhesion_Out_W12 : Outport  Port=11  VectorParamsAs1DForOutWhenUnconnected=off
  V_BCM_COM_Adhesion_Out_W34 : Outport  Port=12  VectorParamsAs1DForOutWhenUnconnected=off
  V_BCM_COM_Opt_Adhesion_Out_W12 : Outport  Port=13  VectorParamsAs1DForOutWhenUnconnected=off
  V_BCM_COM_Opt_Adhesion_Out_W34 : Outport  Port=14  VectorParamsAs1DForOutWhenUnconnected=off
  wires:
  BUS_CAN_BCM_CCDL_RX/1 -> Bus Selector/1
  Mux/1 -> V_BCM_COM_Big_Gamma_Trig_Out_W12/1
  Mux1/1 -> V_BCM_COM_Big_Gamma_Trig_Out_W34/1
  Mux2/1 -> V_BCM_COM_Big_Slip_Trig_Out_W12/1
  Mux3/1 -> V_BCM_COM_Big_Slip_Trig_Out_W34/1
  Mux4/1 -> V_BCM_COM_Big_Slip_WD_In_Mon_W12/1
  Mux5/1 -> V_BCM_COM_Big_Slip_WD_In_Mon_W34/1
  Mux6/1 -> V_BCM_COM_Small_Slip_Trig_Out_W12/1
  Mux7/1 -> V_BCM_COM_Small_Slip_Trig_Out_W34/1
  Mux8/1 -> V_BCM_COM_Target_Speed_Out_W12/1
  Mux9/1 -> V_BCM_COM_Target_Speed_Out_W34/1
  Mux10/1 -> V_BCM_COM_Adhesion_Out_W12/1
  Mux11/1 -> V_BCM_COM_Adhesion_Out_W34/1
  Mux12/1 -> V_BCM_COM_Opt_Adhesion_Out_W12/1
  Mux13/1 -> V_BCM_COM_Opt_Adhesion_Out_W34/1
  Bus Selector/1 -> Mux/1  "<BUS_CAN_BCM_CCDL_TX_V_BCM_COM_Big_Gamma_Trig_Out_W1>"
  Bus Selector/2 -> Mux/2  "<BUS_CAN_BCM_CCDL_TX_V_BCM_COM_Big_Gamma_Trig_Out_W2>"
  Bus Selector/3 -> Mux1/1  "<BUS_CAN_BCM_CCDL_TX_V_BCM_COM_Big_Gamma_Trig_Out_W3>"
  Bus Selector/4 -> Mux1/2  "<BUS_CAN_BCM_CCDL_TX_V_BCM_COM_Big_Gamma_Trig_Out_W4>"
  Bus Selector/5 -> Mux2/1  "<BUS_CAN_BCM_CCDL_TX_V_BCM_COM_Big_Slip_Trig_Out_W1>"
  Bus Selector/6 -> Mux2/2  "<BUS_CAN_BCM_CCDL_TX_V_BCM_COM_Big_Slip_Trig_Out_W2>"
  Bus Selector/7 -> Mux3/1  "<BUS_CAN_BCM_CCDL_TX_V_BCM_COM_Big_Slip_Trig_Out_W3>"
  Bus Selector/8 -> Mux3/2  "<BUS_CAN_BCM_CCDL_TX_V_BCM_COM_Big_Slip_Trig_Out_W4>"
  Bus Selector/9 -> Mux4/1  "<BUS_CAN_BCM_CCDL_TX_V_BCM_COM_Big_Slip_WD_Trig_Out_W1>"
  Bus Selector/10 -> Mux4/2  "<BUS_CAN_BCM_CCDL_TX_V_BCM_COM_Big_Slip_WD_Trig_Out_W2>"
  Bus Selector/11 -> Mux5/1  "<BUS_CAN_BCM_CCDL_TX_V_BCM_COM_Big_Slip_WD_Trig_Out_W3>"
  Bus Selector/12 -> Mux5/2  "<BUS_CAN_BCM_CCDL_TX_V_BCM_COM_Big_Slip_WD_Trig_Out_W4>"
  Bus Selector/13 -> Mux6/1  "<BUS_CAN_BCM_CCDL_TX_V_BCM_COM_Small_Slip_Trig_Out_W1>"
  Bus Selector/14 -> Mux6/2  "<BUS_CAN_BCM_CCDL_TX_V_BCM_COM_Small_Slip_Trig_Out_W2>"
  Bus Selector/15 -> Mux7/1  "<BUS_CAN_BCM_CCDL_TX_V_BCM_COM_Small_Slip_Trig_Out_W3>"
  Bus Selector/16 -> Mux7/2  "<BUS_CAN_BCM_CCDL_TX_V_BCM_COM_Small_Slip_Trig_Out_W4>"
  Bus Selector/17 -> Mux8/1  "<BUS_CAN_BCM_CCDL_TX_V_BCM_COM_Target_Speed_Out_W1>"
  Bus Selector/18 -> Mux8/2  "<BUS_CAN_BCM_CCDL_TX_V_BCM_COM_Target_Speed_Out_W2>"
  Bus Selector/19 -> Mux9/1  "<BUS_CAN_BCM_CCDL_TX_V_BCM_COM_Target_Speed_Out_W3>"
  Bus Selector/20 -> Mux9/2  "<BUS_CAN_BCM_CCDL_TX_V_BCM_COM_Target_Speed_Out_W4>"
  Bus Selector/21 -> Mux10/1  "<BUS_CAN_BCM_CCDL_TX_V_BCM_COM_Adhesion_Out_W1>"
  Bus Selector/22 -> Mux10/2  "<BUS_CAN_BCM_CCDL_TX_V_BCM_COM_Adhesion_Out_W2>"
  Bus Selector/23 -> Mux11/1  "<BUS_CAN_BCM_CCDL_TX_V_BCM_COM_Adhesion_Out_W3>"
  Bus Selector/24 -> Mux11/2  "<BUS_CAN_BCM_CCDL_TX_V_BCM_COM_Adhesion_Out_W4>"
  Bus Selector/25 -> Mux12/1  "<BUS_CAN_BCM_CCDL_TX_V_BCM_COM_Opt_Adhesion_Out_W1>"
  Bus Selector/26 -> Mux12/2  "<BUS_CAN_BCM_CCDL_TX_V_BCM_COM_Opt_Adhesion_Out_W2>"
  Bus Selector/27 -> Mux13/1  "<BUS_CAN_BCM_CCDL_TX_V_BCM_COM_Opt_Adhesion_Out_W3>"
  Bus Selector/28 -> Mux13/2  "<BUS_CAN_BCM_CCDL_TX_V_BCM_COM_Opt_Adhesion_Out_W4>"

== system MATLAB_TEST/AVIONICS/Brake_Control_Module_Side_A/BCSA Controller CP/BUS_CAN_BCM_CCDL_TX ==
  V_BCM_COM_Big_Gamma_Trig_Out_W12 : Inport
  V_BCM_COM_Big_Gamma_Trig_Out_W34 : Inport  Port=2
  V_BCM_COM_Big_Slip_Trig_Out_W12 : Inport  Port=3
  V_BCM_COM_Big_Slip_Trig_Out_W34 : Inport  Port=4
  V_BCM_COM_Big_Slip_WD_Trig_Out_W12 : Inport  Port=5
  V_BCM_COM_Big_Slip_WD_Trig_Out_W34 : Inport  Port=6
  V_BCM_COM_Small_Slip_Trig_Out_W12 : Inport  Port=7
  V_BCM_COM_Small_Slip_Trig_Out_W34 : Inport  Port=8
  V_BCM_COM_Target_Speed_Out_W12 : Inport  Port=9
  V_BCM_COM_Target_Speed_Out_W34 : Inport  Port=10
  V_BCM_COM_Adhesion_Out_W12 : Inport  Port=11
  V_BCM_COM_Adhesion_Out_W34 : Inport  Port=12
  V_BCM_COM_Opt_Adhesion_Out_W12 : Inport  Port=13
  V_BCM_COM_Opt_Adhesion_Out_W34 : Inport  Port=14
  Bus Creator : BusCreator  Inputs=28  OutDataTypeStr=Bus: SMLK_BUS_CAN_BCM_CCDL  NonVirtualBus=on
      settings: InheritFromInputs=off
  Demux{,1..13} (14 alike) : Demux  Outputs=2
  BUS_CAN_BCM_CCDL : Outport  VectorParamsAs1DForOutWhenUnconnected=off
  wires:
  Demux7/2 -> Bus Creator/16  "BUS_CAN_BCM_CCDL_TX_V_BCM_COM_Small_Slip_Trig_Out_W4"
  Demux/1 -> Bus Creator/1  "BUS_CAN_BCM_CCDL_TX_V_BCM_COM_Big_Gamma_Trig_Out_W1"
  Demux9/1 -> Bus Creator/19  "BUS_CAN_BCM_CCDL_TX_V_BCM_COM_Target_Speed_Out_W3"
  Demux8/2 -> Bus Creator/18  "BUS_CAN_BCM_CCDL_TX_V_BCM_COM_Target_Speed_Out_W2"
  V_BCM_COM_Big_Gamma_Trig_Out_W12/1 -> Demux/1  "BUS_CAN_BCM_CCDL_TX_V_BCM_COM_Big_Gamma_Trig_Out_W12"
  V_BCM_COM_Small_Slip_Trig_Out_W12/1 -> Demux6/1  "BUS_CAN_BCM_CCDL_TX_V_BCM_COM_Small_Slip_Trig_Out_W12"
  Demux12/2 -> Bus Creator/26  "BUS_CAN_BCM_CCDL_TX_V_BCM_COM_Opt_Adhesion_Out_W2"
  Demux13/2 -> Bus Creator/28  "BUS_CAN_BCM_CCDL_TX_V_BCM_COM_Opt_Adhesion_Out_W4"
  Demux8/1 -> Bus Creator/17  "BUS_CAN_BCM_CCDL_TX_V_BCM_COM_Target_Speed_Out_W1"
  V_BCM_COM_Big_Gamma_Trig_Out_W34/1 -> Demux1/1  "BUS_CAN_BCM_CCDL_TX_V_BCM_COM_Big_Gamma_Trig_Out_W34"
  Demux11/1 -> Bus Creator/23  "BUS_CAN_BCM_CCDL_TX_V_BCM_COM_Adhesion_Out_W3"
  V_BCM_COM_Target_Speed_Out_W34/1 -> Demux9/1  "BUS_CAN_BCM_CCDL_TX_V_BCM_COM_Target_Speed_Out_W34"
  V_BCM_COM_Small_Slip_Trig_Out_W34/1 -> Demux7/1  "BUS_CAN_BCM_CCDL_TX_V_BCM_COM_Small_Slip_Trig_Out_W34"
  Demux5/1 -> Bus Creator/11  "BUS_CAN_BCM_CCDL_TX_V_BCM_COM_Big_Slip_WD_Trig_Out_W3"
  Demux11/2 -> Bus Creator/24  "BUS_CAN_BCM_CCDL_TX_V_BCM_COM_Adhesion_Out_W4"
  V_BCM_COM_Adhesion_Out_W34/1 -> Demux11/1  "BUS_CAN_BCM_CCDL_TX_V_BCM_COM_Adhesion_Out_W34"
  V_BCM_COM_Target_Speed_Out_W12/1 -> Demux8/1  "BUS_CAN_BCM_CCDL_TX_V_BCM_COM_Target_Speed_Out_W12"
  V_BCM_COM_Big_Slip_Trig_Out_W12/1 -> Demux2/1  "BUS_CAN_BCM_CCDL_TX_V_BCM_COM_Big_Slip_Trig_Out_W12"
  Demux10/2 -> Bus Creator/22  "BUS_CAN_BCM_CCDL_TX_V_BCM_COM_Adhesion_Out_W2"
  V_BCM_COM_Big_Slip_WD_Trig_Out_W12/1 -> Demux4/1  "BUS_CAN_BCM_CCDL_TX_V_BCM_COM_Big_Slip_WD_Trig_Out_W12"
  Demux1/1 -> Bus Creator/3  "BUS_CAN_BCM_CCDL_TX_V_BCM_COM_Big_Gamma_Trig_Out_W3"
  Demux1/2 -> Bus Creator/4  "BUS_CAN_BCM_CCDL_TX_V_BCM_COM_Big_Gamma_Trig_Out_W4"
  Demux12/1 -> Bus Creator/25  "BUS_CAN_BCM_CCDL_TX_V_BCM_COM_Opt_Adhesion_Out_W1"
  Demux9/2 -> Bus Creator/20  "BUS_CAN_BCM_CCDL_TX_V_BCM_COM_Target_Speed_Out_W4"
  V_BCM_COM_Big_Slip_Trig_Out_W34/1 -> Demux3/1  "BUS_CAN_BCM_CCDL_TX_V_BCM_COM_Big_Slip_Trig_Out_W34"
  Demux13/1 -> Bus Creator/27  "BUS_CAN_BCM_CCDL_TX_V_BCM_COM_Opt_Adhesion_Out_W3"
  Demux4/1 -> Bus Creator/9  "BUS_CAN_BCM_CCDL_TX_V_BCM_COM_Big_Slip_WD_Trig_Out_W1"
  V_BCM_COM_Big_Slip_WD_Trig_Out_W34/1 -> Demux5/1  "BUS_CAN_BCM_CCDL_TX_V_BCM_COM_Big_Slip_WD_Trig_Out_W34"
  V_BCM_COM_Opt_Adhesion_Out_W12/1 -> Demux12/1  "BUS_CAN_BCM_CCDL_TX_V_BCM_COM_Opt_Adhesion_Out_W12"
  V_BCM_COM_Opt_Adhesion_Out_W34/1 -> Demux13/1  "BUS_CAN_BCM_CCDL_TX_V_BCM_COM_Opt_Adhesion_Out_W34"
  Demux5/2 -> Bus Creator/12  "BUS_CAN_BCM_CCDL_TX_V_BCM_COM_Big_Slip_WD_Trig_Out_W4"
  V_BCM_COM_Adhesion_Out_W12/1 -> Demux10/1  "BUS_CAN_BCM_CCDL_TX_V_BCM_COM_Adhesion_Out_W12"
  Demux2/2 -> Bus Creator/6  "BUS_CAN_BCM_CCDL_TX_V_BCM_COM_Big_Slip_Trig_Out_W2"
  Demux3/2 -> Bus Creator/8  "BUS_CAN_BCM_CCDL_TX_V_BCM_COM_Big_Slip_Trig_Out_W4"
  Demux3/1 -> Bus Creator/7  "BUS_CAN_BCM_CCDL_TX_V_BCM_COM_Big_Slip_Trig_Out_W3"
  Demux6/1 -> Bus Creator/13  "BUS_CAN_BCM_CCDL_TX_V_BCM_COM_Small_Slip_Trig_Out_W1"
  Demux6/2 -> Bus Creator/14  "BUS_CAN_BCM_CCDL_TX_V_BCM_COM_Small_Slip_Trig_Out_W2"
  Demux7/1 -> Bus Creator/15  "BUS_CAN_BCM_CCDL_TX_V_BCM_COM_Small_Slip_Trig_Out_W3"
  Demux10/1 -> Bus Creator/21  "BUS_CAN_BCM_CCDL_TX_V_BCM_COM_Adhesion_Out_W1"
  Demux/2 -> Bus Creator/2  "BUS_CAN_BCM_CCDL_TX_V_BCM_COM_Big_Gamma_Trig_Out_W2"
  Demux4/2 -> Bus Creator/10  "BUS_CAN_BCM_CCDL_TX_V_BCM_COM_Big_Slip_WD_Trig_Out_W2"
  Bus Creator/1 -> BUS_CAN_BCM_CCDL/1
  Demux2/1 -> Bus Creator/5  "BUS_CAN_BCM_CCDL_TX_V_BCM_COM_Big_Slip_Trig_Out_W1"
